simulink subsystem "VCM_main"  (R2021b)
settings: Solver=VariableStepAuto  StartTime=0.0  StopTime=10.0  RelTol=1e-3
undefined symbols (not defined in the file): df, dr, g, gear_f, gear_r, Iwf, Iwr, l, lf, M, Rwf, Rwr
libraries: simulink x47, dspstat3 x2, dspswit3 x1
(part 4 of 4)

== matlab function VCM_main/TrqClc ==
  data: MaxTorque input; Trq_f output; Trq_r output; CoastTorque input; ReGenerationOn input; ReGenerativeTorque_F input; ReGenerativeTorque_R input; TorqueZeroPosi input; APPS input; APPS output


function [Trq_f, Trq_r, APPS] = fcn(MaxTorque, CoastTorque, ReGenerationOn, ReGenerativeTorque_F, ReGenerativeTorque_R, TorqueZeroPosi, APPS)
    % Linear
    if APPS>=TorqueZeroPosi
        Trq_f=MaxTorque*(APPS-TorqueZeroPosi)/(1-TorqueZeroPosi);
        Trq_r=MaxTorque*(APPS-TorqueZeroPosi)/(1-TorqueZeroPosi);
    else
        if ReGenerationOn>1
            Trq_f=ReGenerativeTorque_F*(APPS-0)/(TorqueZeroPosi-0);
            Trq_r=ReGenerativeTorque_R*(APPS-0)/(TorqueZeroPosi-0);
        else
            Trq_f=-CoastTorque*(APPS-0)/(TorqueZeroPosi-0);
            Trq_r=-CoastTorque*(APPS-0)/(TorqueZeroPosi-0);
    end

    % A Curve
%     X=10;
%     if APPS>=Free
%         Trq=Max*(X^((APPS-Free)/(1-Free))-1)/(X-1);
%     else
%         Trq=0;
%     end
end

== matlab function VCM_main/VDC/DYC1/DYC main/DYC ecopa spec/DYC mode2/DYC Trq ==
  data: RR output; RL output; FR output; TrqF input; TrqR input; KF input; KR input; M input; FL output; delta input; lf parameter; df parameter
function [RR, RL, FR, FL] = fcn(TrqF, TrqR, KF, KR, M, delta, lf, df)
    FL=(1+2*lf/df*tan(delta))*TrqF-(KF*M)/(df*cos(delta));
    FR=(1-2*lf/df*tan(delta))*TrqF+(KF*M)/(df*cos(delta));
    RL=TrqR-(KR*M)/df;
    RR=TrqR+(KR*M)/df;
end

== matlab function VCM_main/VDC/DYC1/DYC main/DYC ecopa spec/DYC mode2/Target Moment ==
  data: a input; Km input; A input; Kfb input; K output; TargetYawRate output; V input; GyroZ input; deltaFB input; deltaFF input; M output; l parameter
function [K, TargetYawRate, M] = fcn(a, Km, A, Kfb, V, GyroZ, deltaFB, deltaFF, l)
    if V<3/3.6
        K=0;
        TargetYawRate=0;
        M=0;
    else
        x0=(Km/2/a + 40)/3.6;
        K=Km*(1/(1+exp(a*(V-x0))));
        Kfb=Kfb*(1/(1+exp(a*(V-x0))));
        TargetYawRate=(1/(1+A*V*V))*(V/l)*deltaFB;
        M=K*deltaFF+Kfb*(TargetYawRate-GyroZ);
    end
end

== stateflow chart VCM_main/VDC/Launch/Chart ==
  state Base
    entry:
    LaunchTorqueLimit = MaxTorqueLimit;
    LaunchLED = 0;
  state OFF
    entry:
    LaunchTorqueLimit = 0;
  state LaunchReady
    entry:
    LaunchTorqueLimit = MaxTorqueLimit;
  state LaunchReady_BrakeON
    entry:
    LaunchTorqueLimit = 0;
    LaunchLED = 1;
  state LaunchReady_BrakeOff
    entry:
    LaunchTorqueLimit = 0;
    state LaunchLEDon
      entry:
      LaunchLED = 1;
    state LaunchLEDoff
      entry:
      LaunchLED = 0;
    (default) -> LaunchLEDon
    LaunchLEDoff -> LaunchLEDon : after(0.2,sec)
    LaunchLEDon -> LaunchLEDoff : after(0.2,sec)
  state LaunchGearProtection
    entry:
    LaunchTorqueLimit = GearProtectionTorqueLimit;
    LaunchLED = 1;
  (default) -> Base
  OFF -> Base : [Torque< 0.5]
  LaunchGearProtection -> Base : after(GearProtectionTime,sec)
  (junction 24) -> OFF
  Base -> LaunchReady : [LaunchSW == 1 & BrakeSW == 1 & rpm < 10 & Torque < 0.3]
  LaunchReady -> (junction 24) [order 2] : [LaunchSW == 0]
  (junction 17) -> (junction 24)
  LaunchReady -> LaunchReady_BrakeON [order 1] : after(2,sec)[BrakeSW == 1]
  LaunchReady_BrakeON -> (junction 17) [order 1] : [LaunchSW == 0]
  LaunchReady_BrakeON -> LaunchReady_BrakeOff [order 2] : after(1,sec)[BrakeSW == 0 & Torque > 5 ]
  LaunchReady_BrakeOff -> LaunchReady_BrakeON [order 1] : [Torque < 4 | BrakeSW == 1]
  LaunchReady_BrakeOff -> LaunchGearProtection [order 2] : [LaunchSW == 0]
  data: LaunchSW input; BrakeSW input; rpm input; Torque input; MaxTorqueLimit input; GearProtectionTorqueLimit input; GearProtectionTime input; LaunchLED output; LaunchTorqueLimit output

== matlab function VCM_main/VDC/DYC1/DYC main/DYC mode1/DYC mode1/DYC Trq ==
  data: RR output; RL output; FR output; TrqF input; TrqR input; KF input; KR input; M input; FL output; delta input; lf parameter; df parameter; DYCtrq output
function [RR, RL, FR, FL,DYCtrq] = fcn(TrqF, TrqR, KF, KR, M, delta, lf, df)

    FL=(1+2*lf/df*tan(delta))*TrqF-(KF*M)/(df*cos(delta));
    FR=(1-2*lf/df*tan(delta))*TrqF+(KF*M)/(df*cos(delta));
    RL=TrqR-(KR*M)/df;
    RR=TrqR+(KR*M)/df;
    DYCtrq = KR*M/df;
end
